simulink model "Tank_Con_Relay"  (R2024b)
settings: Solver=ode45  StartTime=0.0  StopTime=3600  RelTol=1e-3
values from neighbouring files (symbols this model uses):
  A1 = 1.5    [init.m]
  A2 = 1.5    [init.m]
  A3 = 1.5    [init.m]
  h1_0 = 0.4    [init.m]
  h2_0 = 0.3    [init.m]
  h3_0 = 0.2    [init.m]
  k_drain = 0.03    [init.m]
undefined symbols (not defined in the file or in its folder): T1, T3
libraries: slpidlib x1
settings Model: Creator=fatjonkabali  LastModifiedBy=fatjonkabali

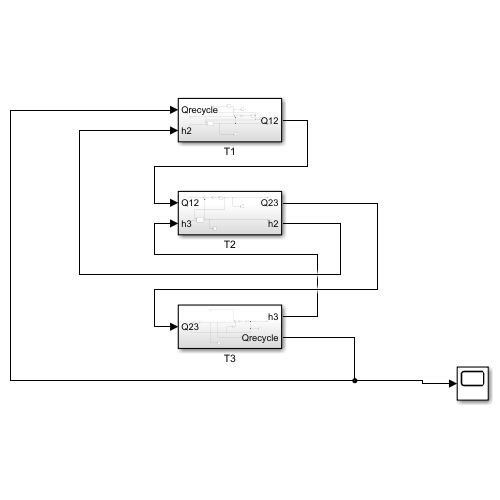
[thumbnail: Simulink's stored preview of the top-level diagram]
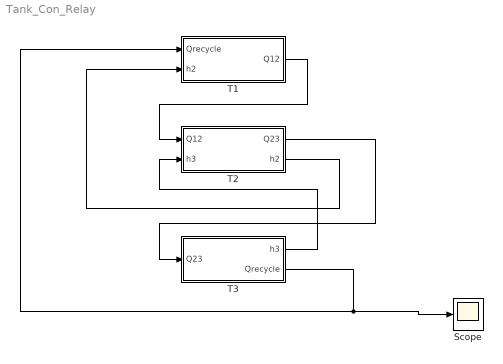
== system Tank_Con_Relay ==
  Scope : Scope
  T1 : Subsystem
  T2 : Subsystem
  T3 : Subsystem
  wires:
  T1/1(Q12) -> T2/1(Q12)
  T2/1(Q23) -> T3/1(Q23)
  T2/2(h2) -> T1/2(h2)
  T3/1(h3) -> T2/2(h3)
  T3/2(Qrecycle) -> Scope/1, T1/1(Qrecycle)

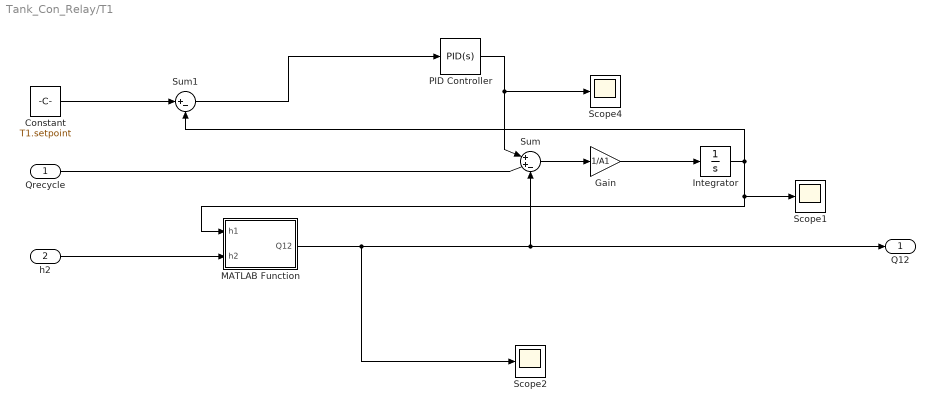
== system Tank_Con_Relay/T1 ==
  Qrecycle : Inport
  h2 : Inport  Port=2
  Constant : Constant  Value=T1.setpoint
  Gain : Gain  Gain=1/A1
  Integrator : Integrator  InitialCondition=h1_0
  MATLAB Function : MATLAB Function  TreatAsAtomicUnit=on
  PID Controller : slpidlib/PID Controller  Controller=PID  Form=Parallel  TimeDomain=Continuous-time  UseExternalTs=off  SampleTime=-1  IntegratorMethod=Forward Euler  FilterMethod=Forward Euler  ControllerParametersSource=internal  P=0.1  I=0.01  UseKiTs=off  D=0.05  UseExternalDerivativeSource=off  N=0  UseFilter=on  TunerSelectOption=Transfer Function Based (PID Tuner App)  InitialConditionSource=internal  InitialConditionForIntegrator=0  InitialConditionForFilter=0  DifferentiatorICPrevScaledInput=0  ExternalReset=none  TrackingMode=off  Kt=1  LimitOutput=on  SatLimitsSource=internal  UpperSaturationLimit=0.5  LowerSaturationLimit=0  LinearizeAsGain=on  AntiWindupMode=none  Kb=1  LimitIntegrator=off  UpperIntegratorSaturationLimit=inf  LowerIntegratorSaturationLimit=-inf  POutMin=[]  POutMax=[]  IOutMin=[]  IOutMax=[]  DOutMin=[]  DOutMax=[]  NOutMin=[]  NOutMax=[]  SumOutMin=[]  SumOutMax=[]  SaturationOutMin=[]  SaturationOutMax=[]  PParamMin=[]  PParamMax=[]  IParamMin=[]  IParamMax=[]  DParamMin=[]  DParamMax=[]  NParamMin=[]  NParamMax=[]  KbParamMin=[]  KbParamMax=[]  KtParamMin=[]  KtParamMax=[]  KbOutMin=[]  KbOutMax=[]  KtOutMin=[]  KtOutMax=[]  IntegratorOutMin=[]  IntegratorOutMax=[]  FilterOutMin=[]  FilterOutMax=[]  SumI1OutMin=[]  SumI1OutMax=[]  SumI2OutMin=[]  SumI2OutMax=[]  SumI3OutMin=[]  SumI3OutMax=[]  SumI4OutMin=[]  SumI4OutMax=[]  SumDOutMin=[]  SumDOutMax=[]  DifferentiatorOutMin=[]  DifferentiatorOutMax=[]  FilterDiffOutCoefMin=[]  FilterDiffOutCoefMax=[]  ReciprocalOutMin=[]  ReciprocalOutMax=[]  SumDenOutMin=[]  SumDenOutMax=[]  SumNumOutMin=[]  SumNumOutMax=[]  DivideOutMin=[]  DivideOutMax=[]  UdiffTsProdOutMin=[]  UdiffTsProdOutMax=[]  NTsProdOutMin=[]  NTsProdOutMax=[]  UintegralTsProdOutMin=[]  UintegralTsProdOutMax=[]  UngainTsProdOutMin=[]  UngainTsProdOutMax=[]  ClampingZeroOutDataTypeStr=Inherit: Inherit via back propagation  ClampingZeroOutMin=[]  ClampingZeroOutMax=[]  FilterDenConstantOutDataTypeStr=Inherit: Inherit via back propagation  FilterDenConstantOutMin=[]  FilterDenConstantOutMax=[]  PCopyOutDataTypeStr=Inherit: Inherit via back propagation  PCopyOutMin=[]  PCopyOutMax=[]  NCopyOutDataTypeStr=Inherit: Inherit via back propagation  NCopyOutMin=[]  NCopyOutMax=[]  IntegratorContinuousStateAttributes=''  IntegratorStateMustResolveToSignalObject=off  IntegratorRTWStateStorageClass=Auto  FilterContinuousStateAttributes=''  FilterStateMustResolveToSignalObject=off  FilterRTWStateStorageClass=Auto  ParallelPVariant=InternalParameters  IdealPVariant=Disabled  IVariant=InternalParameters  DVariant=InternalParameters  IntegratorVariant=Continuous  SatVariant=Enabled  AWVariant=Passthrough  PCopyVariant=Disabled  TRVariant=Disabled  FdbkBlocksVariant=Forward  IdealPFdbkVariant=Disabled  SatFdbkVariant=Disabled  DerivativeFilterVariant=ContFilter  NVariant=InternalParameters  NCopyVariant=Disabled  FilterICVariant=InternalICsFilter  IntegratorICVariant=InternalICs  ExternalResetVariant=Disabled  TRSumVariant=Passthrough  SumFdbkVariant=Disabled  SumVariant=Sum_PID  TsampFilterVariant=InternalTs  TsampNgainVariant=Passthrough  TsampIntegralVariant=Disabled_SignalSpec  ExternalSaturationOutDataTypeStr=Inherit: Same as second input  DerivativeSourceVariant=ErrorSignal  PreIntVariant=InternalPreInt
  Scope1 : Scope
  Scope2 : Scope
  Scope4 : Scope
  Sum : Sum  Inputs=|++-
  Sum1 : Sum  Inputs=|+-
  Q12 : Outport
  wires:
  MATLAB Function/1(Q12) -> Scope2/1, Sum/3, Q12/1
  Qrecycle/1 -> Sum/2
  PID Controller/1 -> Scope4/1, Sum/1
  Sum/1 -> Gain/1
  Gain/1 -> Integrator/1
  Integrator/1 -> Sum1/2, Scope1/1, MATLAB Function/1(h1)
  h2/1 -> MATLAB Function/2(h2)
  Sum1/1 -> PID Controller/1
  Constant/1 -> Sum1/1

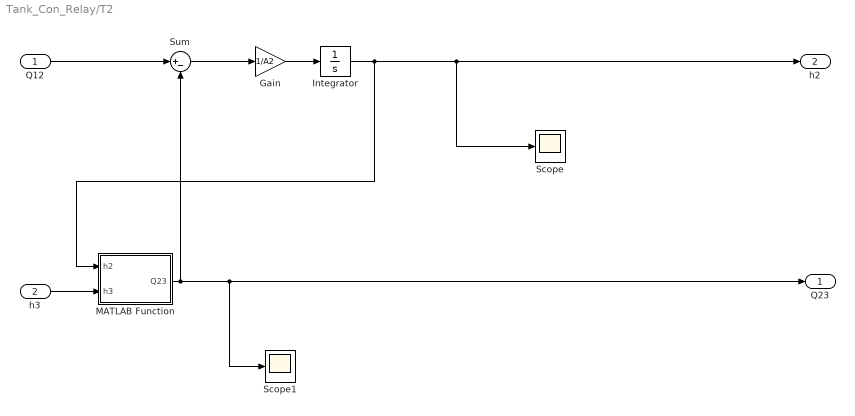
== system Tank_Con_Relay/T2 ==
  Q12 : Inport
  h3 : Inport  Port=2
  Gain : Gain  Gain=1/A2
  Integrator : Integrator  InitialCondition=h2_0
  MATLAB Function : MATLAB Function  TreatAsAtomicUnit=on
  Scope : Scope
  Scope1 : Scope
  Sum : Sum  Inputs=|+-
  Q23 : Outport
  h2 : Outport  Port=2
  wires:
  Integrator/1 -> MATLAB Function/1(h2), Scope/1, h2/1
  MATLAB Function/1(Q23) -> Scope1/1, Q23/1, Sum/2
  Q12/1 -> Sum/1
  Sum/1 -> Gain/1
  Gain/1 -> Integrator/1
  h3/1 -> MATLAB Function/2(h3)

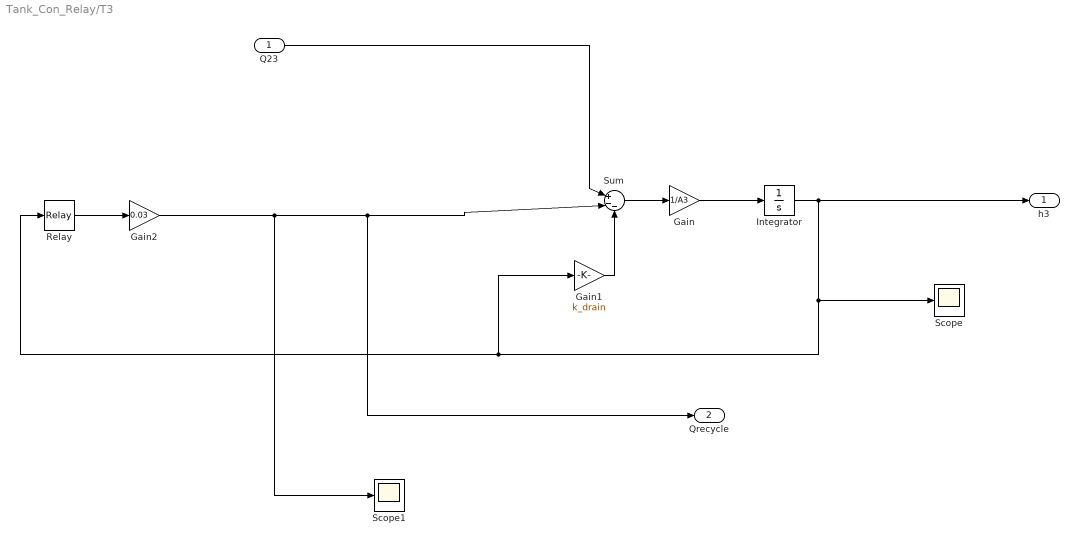
== system Tank_Con_Relay/T3 ==
  Q23 : Inport
  Gain : Gain  Gain=1/A3
  Gain1 : Gain  Gain=k_drain
  Gain2 : Gain  Gain=0.03
  Integrator : Integrator  InitialCondition=h3_0  LowerSaturationLimit=0
  Relay : Relay  OnSwitchValue=T3.setpoint  OffSwitchValue=T3.setpoint-0.0001  OnOutputValue=0.1  ZeroCross=off
  Scope : Scope
  Scope1 : Scope
  Sum : Sum  Inputs=|+--
  h3 : Outport
  Qrecycle : Outport  Port=2
  wires:
  Q23/1 -> Sum/1
  Gain/1 -> Integrator/1
  Sum/1 -> Gain/1
  Gain1/1 -> Sum/3
  Relay/1 -> Gain2/1
  Integrator/1 -> Scope/1, Relay/1, Gain1/1, h3/1
  Gain2/1 -> Qrecycle/1, Sum/2, Scope1/1

== matlab function Tank_Con_Relay/T1/MATLAB Function ==
  data: h1 input; Q12 output; h2 input
function Q12 = flow12(h1, h2)
    k1 = 0.08;
    Q12 = k1 * sign(h1 - h2) * sqrt(abs(h1 - h2));
end

== matlab function Tank_Con_Relay/T2/MATLAB Function ==
  data: h2 input; Q23 output; h3 input
function Q23 = flow23(h2, h3)
    k2 = 0.06;
    Q23 = k2 * sign(h2 - h3) * sqrt(abs(h2 - h3));
end
